simulink model "sampleModel1574_2"  (R2023a)
settings: Solver=VariableStepAuto  StartTime=0.0  StopTime=10.0  RelTol=1e-3
libraries: hdlsllib x5, simulink x3
settings Model: Creator=user1  LastModifiedBy=user1

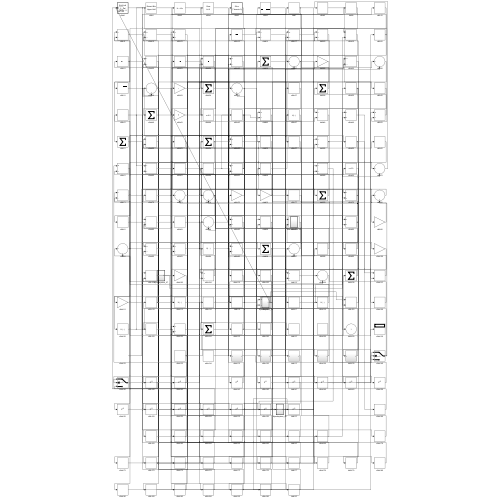
[thumbnail: Simulink's stored preview of the top-level diagram]
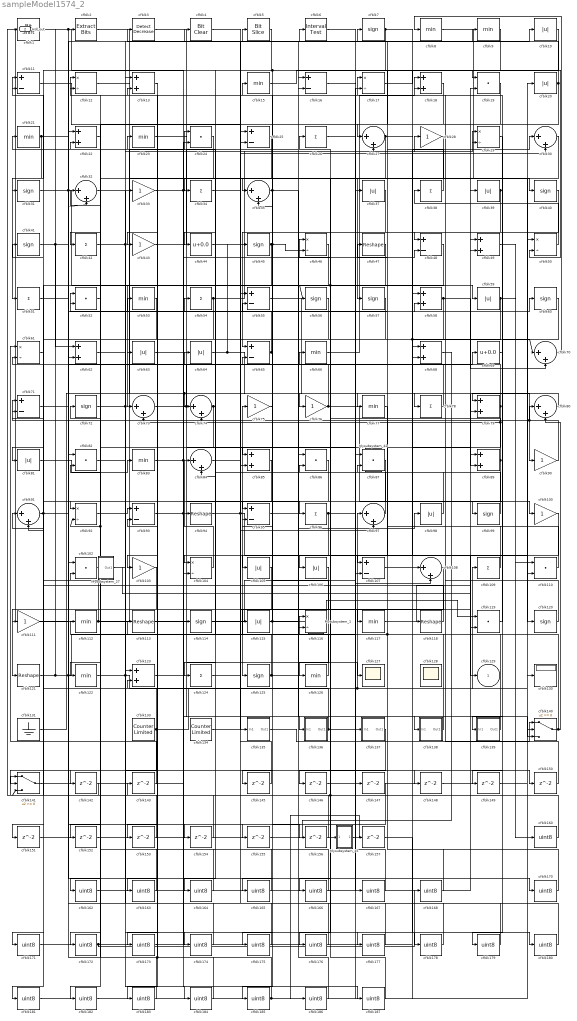
== system sampleModel1574_2 ==
  Mysubsystem_1 : Subsystem  TreatAsAtomicUnit=on  RTWFcnName=Mysubsystem_1
      settings: RTWFcnNameOpts=User specified  RTWFileNameOpts=Use function name
  Mysubsystem_27 : Subsystem  TreatAsAtomicUnit=on  RTWFcnName=Mysubsystem_27
      settings: RTWFcnNameOpts=User specified  RTWFileNameOpts=Use function name
  Mysubsystem_42 : Subsystem  TreatAsAtomicUnit=on  RTWFcnName=Mysubsystem_42
      settings: RTWFcnNameOpts=User specified  RTWFileNameOpts=Use function name
  Mysubsystem_45 : Subsystem  TreatAsAtomicUnit=on  RTWFcnName=Mysubsystem_45
      settings: RTWFcnNameOpts=User specified  RTWFileNameOpts=Use function name
  cfblk1 : hdlsllib/Logic and Bit Operations/Bit Shift  mode=Shift Left Logical  N=0
  cfblk{10,20,37,39,59,63..64,81,98,105..106,115} (12 alike) : Abs  OutDataTypeStr=uint8  SaturateOnIntegerOverflow=off
  cfblk{28,33,43,75..76,90,100,103,111} (9 alike) : Gain  OutDataTypeStr=uint8
  cfblk{19,24,52,82,86..87,102,110,119} (9 alike) : DotProduct  OutDataTypeStr=uint8
  cfblk{12,17,29,46,50,61,92,104,116} (9 alike) : Product  Inputs=*/  OutDataTypeStr=uint8  RndMeth=Zero  SaturateOnIntegerOverflow=on
  cfblk{11,16,25,48,55,65,71,93,95,107} (10 alike) : Sum  Inputs=+-  OutDataTypeStr=uint8
  cfblk{27,30,32,35,70,73..74,80,84,91,97,108} (12 alike) : Sum  Inputs=|++  OutDataTypeStr=uint8
  cfblk{26,34,38,42,51,54,78,96,109,124} (10 alike) : Sum  Inputs=+  OutDataTypeStr=uint8
  cfblk{8..9,15,21,23,53,66,77,83,112,117,122,126} (13 alike) : MinMax  OutDataTypeStr=uint8
  cfblk{47,94,113,118,121} (5 alike) : Reshape
  cfblk{7,31,40..41,45,56..57,60,72,99,114,120,125} (13 alike) : Signum
  cfblk{13,18,22,49,58,62,68,79,85,89,123} (11 alike) : Sum  OutDataTypeStr=uint8
  cfblk127 : Scope
  cfblk128 : Scope
      settings: Floating=on
  cfblk130 : Display
  cfblk131 : Ground
  cfblk133 : hdlsllib/Sources/Counter Limited  uplimit=7  tsamp=-1
  cfblk134 : hdlsllib/Sources/Counter Limited  uplimit=7  tsamp=-1
  cfblk135 : Subsystem
      settings: LibrarySourceBlock=|
      | hdlsllib/Ports &
      | Subsystems/Subsystem
  cfblk136 : Subsystem
      settings: LibrarySourceBlock=|
      | hdlsllib/Ports &
      | Subsystems/Subsystem
  cfblk137 : Subsystem
      settings: LibrarySourceBlock=|
      | hdlsllib/Ports &
      | Subsystems/Subsystem
  cfblk138 : Subsystem
      settings: LibrarySourceBlock=|
      | hdlsllib/Ports &
      | Subsystems/Subsystem
  cfblk139 : Subsystem
      settings: LibrarySourceBlock=|
      | hdlsllib/Ports &
      | Subsystems/Subsystem
  cfblk140 : Switch  OutDataTypeStr=uint8  SaturateOnIntegerOverflow=off  InputSameDT=off
  cfblk141 : Switch  OutDataTypeStr=uint8  SaturateOnIntegerOverflow=off  InputSameDT=off
  cfblk{142..143,145..157} (15 alike) : Delay  SampleTime=1
  cfblk{160,162..168,170..187} (26 alike) : DataTypeConversion  OutDataTypeStr=uint8  SaturateOnIntegerOverflow=off  RndMeth=Floor
  cfblk2 : simulink/Logic and Bit Operations/Extract Bits  bitsToExtract=Upper half  numBits=8  bitIdxRange=[0 7]  outScalingMode=Preserve fixed-point scaling
      settings: LibrarySourceBlock=|
      | hdlsllib/Logic and Bit
      | Operations/Extract Bits
  cfblk3 : simulink/Logic and Bit Operations/Detect Decrease  vinit=0.0  OutDataTypeStr=uint8
      settings: LibrarySourceBlock=|
      | hdlsllib/Logic and Bit
      | Operations/Detect
      | Decrease
  cfblk4 : simulink/Logic and Bit Operations/Bit Clear  iBit=0
      settings: LibrarySourceBlock=|
      | hdlsllib/Logic and Bit
      | Operations/Bit Clear
  cfblk44 : Bias  Bias=0.0  SaturateOnIntegerOverflow=off
  cfblk5 : hdlsllib/Logic and Bit Operations/Bit Slice  lidx=7  ridx=0
  cfblk6 : hdlsllib/Logic and Bit Operations/Interval Test  IntervalClosedRight=on  uplimit=0.5  IntervalClosedLeft=on  lowlimit=-0.5  OutDataTypeStr=uint8
  cfblk69 : Bias  Bias=0.0  SaturateOnIntegerOverflow=off
  cfblk129 : Outport  OutDataTypeStr=uint8  VectorParamsAs1DForOutWhenUnconnected=off
  Hdl_out : Outport  Port=2  OutDataTypeStr=uint8
  wires:
  cfblk122/1 -> cfblk109/1, cfblk69/1
  cfblk140/1 -> cfblk116/1, cfblk80/2
  cfblk133/1 -> cfblk97/1, cfblk20/1, cfblk141/2, cfblk91/2
  cfblk105/1 -> cfblk125/1
  cfblk131/1 -> cfblk76/1
  cfblk119/1 -> cfblk12/1
  cfblk3/1 -> cfblk136/1(In1)
  cfblk44/1 -> cfblk135/1(In1)
  cfblk120/1 -> cfblk71/1
  cfblk42/1 -> cfblk4/1, cfblk178/1
  cfblk112/1 -> cfblk24/1, cfblk91/1
  cfblk48/1 -> cfblk73/1
  cfblk41/1 -> cfblk82/1, cfblk62/1
  cfblk49/1 -> cfblk160/1
  cfblk78/1 -> cfblk11/1
  cfblk2/1 -> cfblk78/1
  cfblk21/1 -> cfblk51/1, cfblk77/1
  cfblk43/1 -> cfblk16/2
  cfblk30/1 -> cfblk106/1, cfblk56/1
  cfblk126/1 -> cfblk75/1
  cfblk15/1 -> cfblk50/2
  cfblk93/1 -> cfblk127/1, cfblk48/2
  cfblk20/1 -> cfblk5/1, cfblk42/1
  cfblk63/1 -> cfblk96/1
  cfblk82/1 -> cfblk33/1
  cfblk116/1 -> cfblk126/1, cfblk95/2
  cfblk16/1 -> cfblk137/1(In1)
  cfblk55/1 -> cfblk90/1
  cfblk25/1 -> cfblk43/1
  cfblk65/1 -> cfblk52/1, cfblk35/2
  cfblk18/1 -> cfblk34/1
  cfblk76/1 -> cfblk100/1, cfblk65/2
  cfblk66/1 -> cfblk18/1
  cfblk80/1 -> cfblk79/1
  cfblk89/1 -> cfblk46/1, cfblk74/2, cfblk151/1
  cfblk23/1 -> cfblk57/1
  cfblk5/1 -> cfblk31/1
  cfblk37/1 -> cfblk85/1
  cfblk95/1 -> cfblk138/1(In1)
  cfblk31/1 -> cfblk59/1, cfblk32/2
  cfblk71/1 -> cfblk66/1
  cfblk98/1 -> cfblk61/2
  cfblk61/1 -> cfblk81/1
  cfblk136/1(Out1) -> cfblk92/2, cfblk12/2, cfblk108/2
  cfblk8/1 -> cfblk40/1
  cfblk54/1 -> cfblk29/1, cfblk62/2
  cfblk53/1 -> cfblk172/1
  cfblk17/1 -> cfblk19/1
  cfblk79/1 -> cfblk92/1, cfblk32/1
  cfblk70/1 -> cfblk8/1
  cfblk40/1 -> cfblk65/1
  cfblk107/1 -> cfblk30/1
  cfblk91/1 -> cfblk11/2, cfblk154/1
  cfblk9/1 -> cfblk44/1, cfblk95/1
  cfblk121/1 -> cfblk37/1, cfblk58/2, cfblk2/1
  cfblk85/1 -> cfblk122/1
  cfblk117/1 -> cfblk39/1
  cfblk125/1 -> cfblk10/1, cfblk93/2
  cfblk135/1(Out1) -> cfblk140/1
  cfblk64/1 -> cfblk89/1, cfblk45/1
  cfblk12/1 -> cfblk120/1
  cfblk104/1 -> cfblk84/1
  cfblk46/1 -> cfblk103/1
  cfblk4/1 -> cfblk117/1
  cfblk110/1 -> cfblk54/1
  cfblk86/1 -> cfblk185/1
  cfblk1/1 -> cfblk74/1, cfblk79/2, cfblk94/1
  cfblk72/1 -> cfblk29/2, cfblk148/1
  cfblk58/1 -> cfblk70/2, cfblk146/1
  cfblk83/1 -> cfblk28/1, cfblk140/3
  cfblk69/1 -> cfblk99/1
  cfblk75/1 -> cfblk15/1
  cfblk99/1 -> cfblk21/1
  cfblk115/1 -> cfblk98/1, cfblk55/2
  cfblk45/1 -> cfblk105/1, cfblk46/2, cfblk111/1
  cfblk118/1 -> cfblk41/1
  cfblk138/1(Out1) -> cfblk52/2
  cfblk100/1 -> cfblk104/1
  cfblk27/1 -> cfblk63/1, cfblk89/2
  cfblk33/1 -> cfblk35/1, cfblk155/1
  cfblk108/1 -> cfblk121/1
  cfblk59/1 -> cfblk124/1, cfblk110/1
  cfblk38/1 -> cfblk3/1
  cfblk7/1 -> cfblk70/1, cfblk110/2, cfblk84/2
  cfblk97/1 -> cfblk73/2
  cfblk77/1 -> cfblk107/1
  cfblk11/1 -> cfblk85/2
  cfblk39/1 -> cfblk139/1(In1), cfblk48/1
  cfblk74/1 -> cfblk164/1, cfblk173/1
  cfblk96/1 -> cfblk104/2, cfblk150/1
  cfblk124/1 -> cfblk7/1
  cfblk34/1 -> cfblk97/2
  cfblk73/1 -> cfblk107/2, cfblk27/2
  cfblk139/1(Out1) -> cfblk17/1, cfblk64/1
  cfblk141/1 -> cfblk114/1
  cfblk81/1 -> cfblk83/1
  cfblk94/1 -> cfblk25/2, cfblk129/1
  cfblk114/1 -> cfblk17/2
  cfblk50/1 -> cfblk38/1
  cfblk92/1 -> cfblk93/1
  cfblk109/1 -> cfblk6/1
  cfblk10/1 -> cfblk27/1
  cfblk35/1 -> cfblk119/2, cfblk165/1
  cfblk57/1 -> cfblk115/1
  cfblk134/1 -> cfblk30/2
  cfblk111/1 -> cfblk9/1
  cfblk84/1 -> cfblk60/1
  cfblk90/1 -> cfblk47/1, cfblk80/1
  cfblk28/1 -> cfblk142/1
  cfblk142/1 -> cfblk1/1
  cfblk143/1 -> cfblk61/1
  cfblk106/1 -> cfblk145/1
  cfblk145/1 -> cfblk25/1
  cfblk146/1 -> cfblk140/2
  cfblk26/1 -> cfblk147/1
  cfblk148/1 -> cfblk19/2
  cfblk29/1 -> cfblk149/1
  cfblk149/1 -> cfblk50/1
  cfblk150/1 -> cfblk18/2
  cfblk151/1 -> cfblk108/1
  cfblk103/1 -> cfblk152/1
  cfblk152/1 -> cfblk116/2
  cfblk24/1 -> cfblk153/1
  cfblk153/1 -> cfblk71/2
  cfblk154/1 -> cfblk141/1
  cfblk155/1 -> cfblk58/1
  cfblk62/1 -> cfblk156/1
  cfblk156/1 -> cfblk16/1
  cfblk160/1 -> cfblk141/3, cfblk26/1
  cfblk52/1 -> cfblk162/1
  cfblk162/1 -> cfblk49/2
  cfblk13/1 -> cfblk163/1
  cfblk163/1 -> cfblk112/1
  cfblk164/1 -> cfblk13/1
  cfblk165/1 -> cfblk13/2
  cfblk87/1 -> cfblk166/1
  cfblk166/1 -> cfblk143/1
  cfblk6/1 -> cfblk167/1
  cfblk167/1 -> cfblk87/1
  cfblk168/1 -> cfblk87/2
  cfblk51/1 -> cfblk170/1
  cfblk170/1 -> cfblk68/1
  cfblk56/1 -> cfblk171/1
  cfblk171/1 -> cfblk68/2
  cfblk172/1 -> cfblk168/1, cfblk24/2
  cfblk173/1 -> cfblk53/1
  cfblk102/1 -> cfblk174/1
  cfblk174/1 -> cfblk113/1
  cfblk147/1 -> cfblk175/1
  cfblk175/1 -> cfblk102/1
  cfblk137/1(Out1) -> cfblk176/1
  cfblk176/1 -> cfblk102/2
  cfblk123/1 -> cfblk177/1
  cfblk177/1 -> cfblk72/1
  cfblk178/1 -> cfblk123/1
  cfblk60/1 -> cfblk179/1
  cfblk179/1 -> cfblk123/2
  cfblk157/1 -> cfblk180/1
  cfblk180/1 -> cfblk55/1
  cfblk47/1 -> cfblk181/1
  cfblk181/1 -> cfblk157/1
  cfblk22/1 -> cfblk182/1
  cfblk182/1 -> cfblk118/1
  cfblk19/1 -> cfblk183/1
  cfblk183/1 -> cfblk22/1
  cfblk32/1 -> cfblk184/1
  cfblk184/1 -> cfblk22/2
  cfblk185/1 -> cfblk82/2, cfblk23/1, cfblk130/1
  cfblk186/1 -> cfblk86/1
  cfblk113/1 -> cfblk187/1
  cfblk187/1 -> cfblk86/2
  Mysubsystem_1/1(Out1) -> cfblk119/1, Hdl_out/1
  Mysubsystem_27/1(Out1) -> cfblk49/1
  cfblk68/1 -> Mysubsystem_45/1(In1)
  Mysubsystem_45/1(Out1) -> cfblk186/1

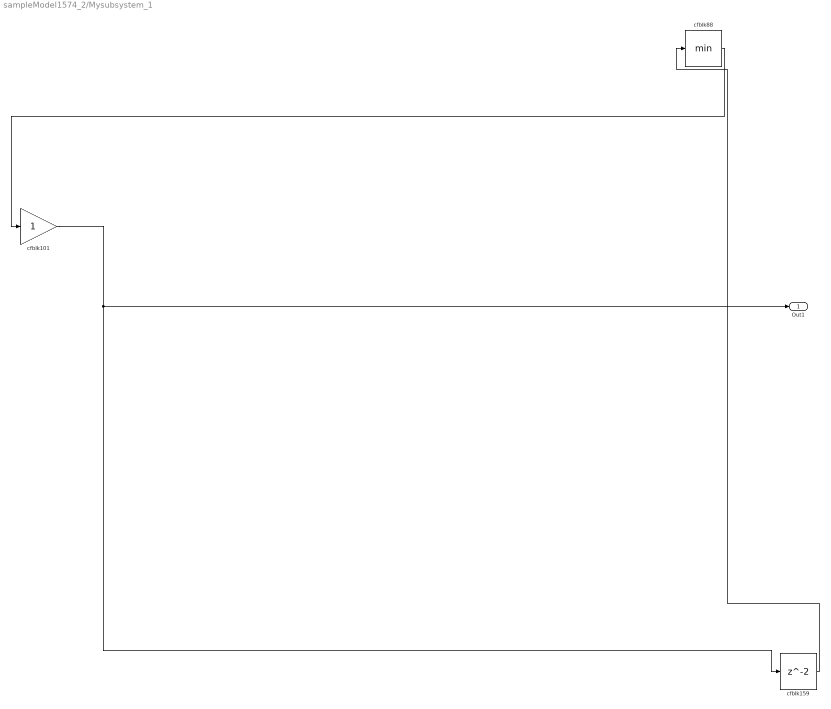
== system sampleModel1574_2/Mysubsystem_1 ==
  cfblk101 : Gain
  cfblk159 : Delay  SampleTime=1
  cfblk88 : MinMax
  Out1 : Outport
  wires:
  cfblk159/1 -> cfblk88/1
  cfblk101/1 -> Out1/1, cfblk159/1
  cfblk88/1 -> cfblk101/1

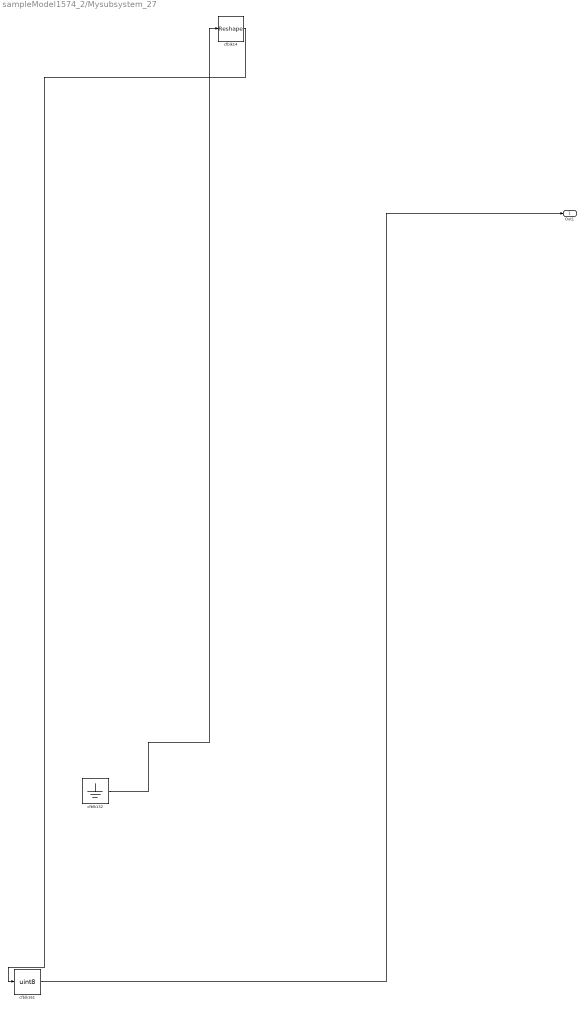
== system sampleModel1574_2/Mysubsystem_27 ==
  cfblk132 : Ground
  cfblk14 : Reshape
  cfblk161 : DataTypeConversion  OutDataTypeStr=uint8  SaturateOnIntegerOverflow=off  RndMeth=Floor
  Out1 : Outport
  wires:
  cfblk14/1 -> cfblk161/1
  cfblk161/1 -> Out1/1
  cfblk132/1 -> cfblk14/1

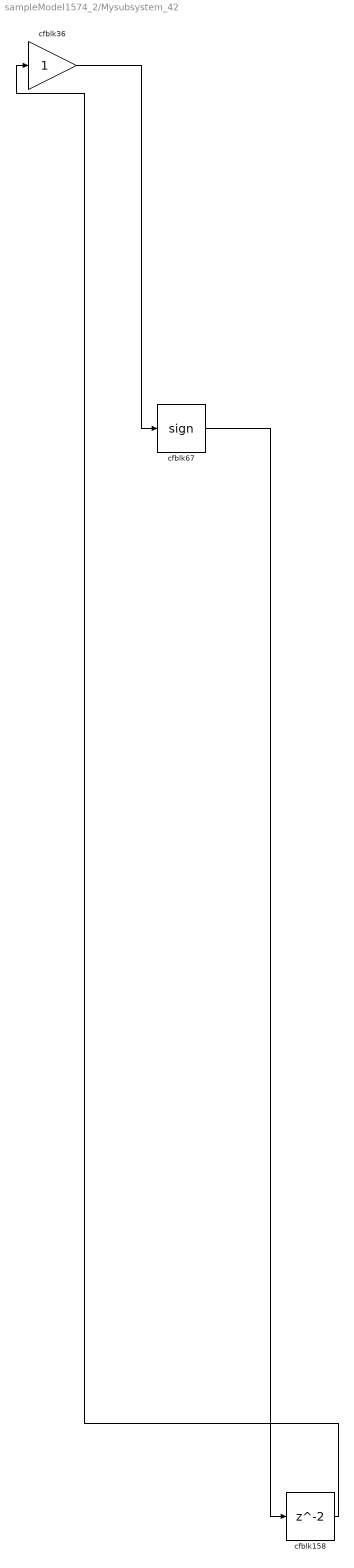
== system sampleModel1574_2/Mysubsystem_42 ==
  cfblk158 : Delay  SampleTime=1
  cfblk36 : Gain
  cfblk67 : Signum
  wires:
  cfblk67/1 -> cfblk158/1
  cfblk158/1 -> cfblk36/1
  cfblk36/1 -> cfblk67/1

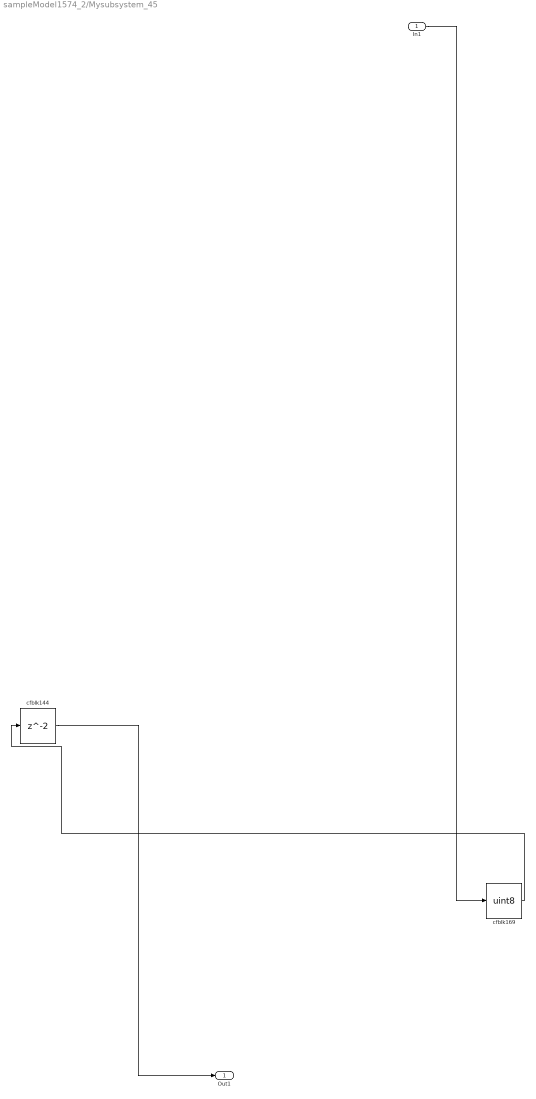
== system sampleModel1574_2/Mysubsystem_45 ==
  In1 : Inport
  cfblk144 : Delay  SampleTime=1
  cfblk169 : DataTypeConversion  OutDataTypeStr=uint8  SaturateOnIntegerOverflow=off  RndMeth=Floor
  Out1 : Outport
  wires:
  In1/1 -> cfblk169/1
  cfblk169/1 -> cfblk144/1
  cfblk144/1 -> Out1/1

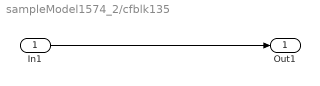
== system sampleModel1574_2/cfblk135 ==
  In1 : Inport
  Out1 : Outport
  wires:
  In1/1 -> Out1/1

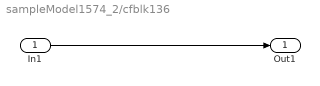
== system sampleModel1574_2/cfblk136 ==
  In1 : Inport
  Out1 : Outport
  wires:
  In1/1 -> Out1/1

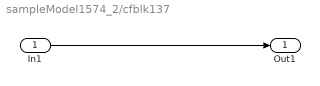
== system sampleModel1574_2/cfblk137 ==
  In1 : Inport
  Out1 : Outport
  wires:
  In1/1 -> Out1/1

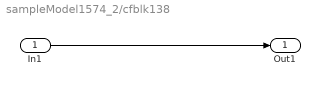
== system sampleModel1574_2/cfblk138 ==
  In1 : Inport
  Out1 : Outport
  wires:
  In1/1 -> Out1/1

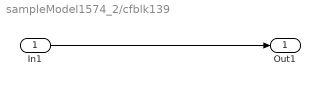
== system sampleModel1574_2/cfblk139 ==
  In1 : Inport
  Out1 : Outport
  wires:
  In1/1 -> Out1/1
